simulink model "PM_fnc20_abs_ampslimit_1Dlookup_TestHarness"  (R2022a)
settings: Solver=VariableStepAuto  StartTime=0.0  StopTime=inf  RelTol=1e-3
settings Model: Creator=306427  LastModifiedBy=306427

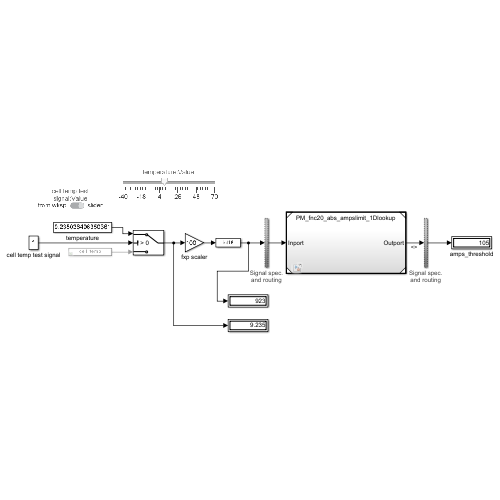
[thumbnail: Simulink's stored preview of the top-level diagram]
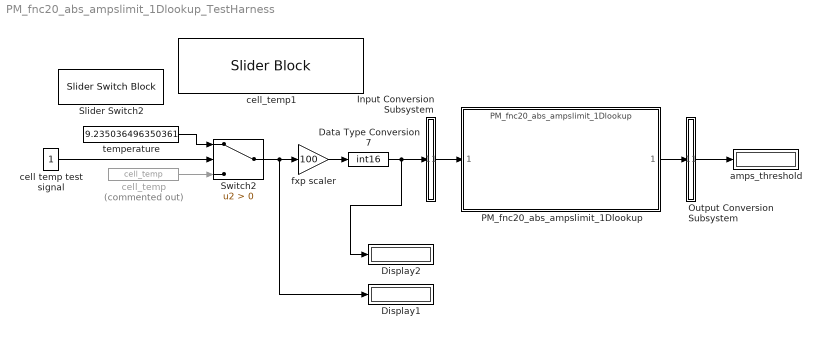
== system PM_fnc20_abs_ampslimit_1Dlookup_TestHarness ==
  Data Type Conversion7 : DataTypeConversion  OutDataTypeStr=int16  SaturateOnIntegerOverflow=off  RndMeth=Floor
  Display1 : Display
  Display2 : Display
  Input Conversion Subsystem : Subsystem  Tag=__SLT_ICS__  Description=|
      | Signal spec.
      | and routing
      settings: AttributesFormatString=%<Description>
  Output Conversion Subsystem : Subsystem  Tag=__SLT_OCS__  Description=|
      | Signal spec.
      | and routing
      settings: AttributesFormatString=%<Description>
  PM_fnc20_abs_ampslimit_1Dlookup : ModelReference  ModelNameDialog=PM_fnc20_abs_ampslimit_1Dlookup  SimulationMode=Normal  ModelReferenceVersion=1.6
  Slider Switch2 : SliderSwitchBlock
      settings: Values={{'from wksp', 'slider'}, [0 1]}
  Switch2 : Switch  Criteria=u2 > Threshold  SaturateOnIntegerOverflow=off  InputSameDT=off
  amps_threshold : Display
  cell temp test signal : Constant
  cell_temp : FromWorkspace  Commented=on  VariableName=cell_temp  OutDataTypeStr=double  SampleTime=[0, 1]
  cell_temp1 : SliderBlock  ScaleMin=-40  ScaleMax=70
  fxp scaler : Gain  Gain=100
  temperature : Constant  Value=9.235036496350361  OutDataTypeStr=double
  wires:
  Input Conversion Subsystem/1(Outport_1) -> PM_fnc20_abs_ampslimit_1Dlookup/1
  PM_fnc20_abs_ampslimit_1Dlookup/1 -> Output Conversion Subsystem/1(Inport_1)
  temperature/1 -> Switch2/1
  cell_temp/1 -> Switch2/3
  Output Conversion Subsystem/1(Outport_1) -> amps_threshold/1
  cell temp test signal/1 -> Switch2/2
  Switch2/1 -> Display1/1, fxp scaler/1
  Data Type Conversion7/1 -> Display2/1, Input Conversion Subsystem/1(Inport_1)
  fxp scaler/1 -> Data Type Conversion7/1

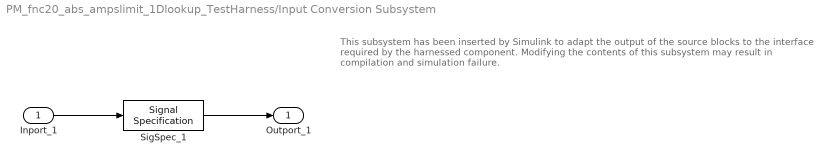
== system PM_fnc20_abs_ampslimit_1Dlookup_TestHarness/Input Conversion Subsystem ==
  note: This subsystem has been inserted by Simulink to adapt the output of the source blocks to the interface required by the harnessed component.
      |  Modifying the contents of this subsystem may result in compilation and simulation failure.
  Inport_1 : Inport
  SigSpec_1 : SignalSpecification  OutDataTypeStr=int16  Dimensions=[1]  SampleTime=[0, 0]
  Outport_1 : Outport
  wires:
  SigSpec_1/1 -> Outport_1/1
  Inport_1/1 -> SigSpec_1/1

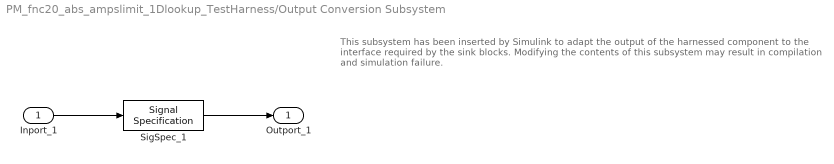
== system PM_fnc20_abs_ampslimit_1Dlookup_TestHarness/Output Conversion Subsystem ==
  note: This subsystem has been inserted by Simulink to adapt the output of the harnessed component to the interface required by the sink blocks.
      |  Modifying the contents of this subsystem may result in compilation and simulation failure.
  Inport_1 : Inport
  SigSpec_1 : SignalSpecification  OutDataTypeStr=int16  Dimensions=[1]
  Outport_1 : Outport
  wires:
  Inport_1/1 -> SigSpec_1/1
  SigSpec_1/1 -> Outport_1/1
